simulink library "SimplusGT_2018b"  (R2018b)
settings: Solver=ode45  StartTime=0.0  StopTime=10.0  RelTol=1e-3
undefined symbols (not defined in the file): ang_r, Cf, DiscIntNeverNeededParam, initial, Lc, Lf, m, OtherInputs, P_dc, Sbase, t0, Tm_pu, Ts, V, Vbase, w_droop, w_i, w_pll, w_tau, w_v, Wbase, wc, wfil, x0, Ybase, Zbase
libraries: powerlib x224, SimplexPS_2015a x6, $bdroot x1
(part 1 of 5)
settings Model: Creator=admin_user  LastModifiedBy=yz34218
settings OptimizationCC: LifeSpan=inf
settings DebuggingCC: SFExecutionAtInitializationDiag=none
settings HardwareCC: ProdBitPerSizeT=32  ProdBitPerPtrDiffT=32  ProdWordSize=32  ProdHWDeviceType=Specified
settings SFSimCC: SimUseLocalCustomCode=off
settings RTWCC: RTWUseLocalCustomCode=off
settings CodeAppCC: StateflowObjectComments=on

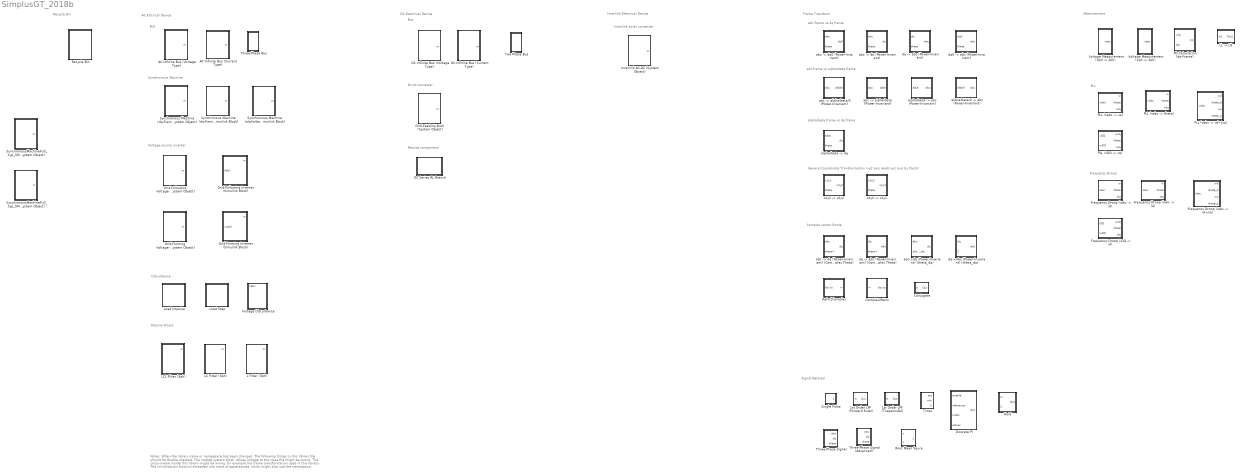
== system SimplusGT_2018b ==
  note: Notes:
      |
      | When the library name or namespace has been changed. The following things in this library file should be double checked.
      |
      | The matlab system block, whose linkage to the class file might be wrong.
      | The cross-invoke inside this library might be wrong, for example the frame transformation used in this library.
      | The initialization function embeded into mask of apparatuses, which might also use the namespace.
  note: Recycle Bin
  note: Interlink ac-dc converter
  note: Interlink Electrical Device
  note: Dc-dc converter:
  note: DC Electrical Device
  note: Passive Filters
  note: alpha/beta frame vs dq frame
  note: Frequency Droop
  note: PLL
  note: Complex vector frame
  note: abc frame vs alpha/beta frame
  note: abc frame vs dq frame
  note: Signal Related
  note: AC Elctrical Device
  note: Measurement
  note: Frame Transform
  note: Bus
  note: Synchronous Machine
  note: Voltage-source inverter
  note: Disturbance
  note: General Coordinate Transformation (xy2 axis leads xy1 axis by theta)
  note: Bus
  note: Passive component:
  1st Order LPF (Forward Euler) : Subsystem  mask{wc=wfil, Ts=Ts}
      mask prompts: wc "wc (rad/s), bandwidth"; Ts "Ts (s), sampling period"
  1st Order LPF (Trapezoidal) : Subsystem  mask{Ts=0, wc=0}
      mask prompts: Ts "Ts (s), sampling period"; wc "wc (rad/s), bandwidth"
  AC Infinite Bus (Current Type) : Subsystem  mask{Ts=Ts, Sbase=Sbase, Vbase=Vbase, Wbase=Wbase, id=1, iq=0, theta0=0, w=1}
      mask prompts: Ts "Ts (s), sampling period"; Sbase "Sbase (VA), base power"; Vbase "Vbase (V), base voltage"; Wbase "Wbase (rad/s), base angular frequency"; id "id (pu), d-axis current"; iq "iq (pu), q-axis current"; theta0 "theta0 (rad), initial angle"; w "w (pu), angular frequency"
  AC Infinite Bus (Voltage Type) : Subsystem  mask{Ts=Ts, Sbase=Sbase, Vbase=Vbase, Wbase=Wbase, vd=1, vq=0, theta0=0, w=Wbase, R=1e-30}
      mask prompts: Ts "Ts (s), samping period"; Sbase "Sbase (VA), power base"; Vbase "Vbase (V), voltage base"; Wbase "Wbase (rad/s), frequency base"; vd "vd (pu), d-axis voltage"; vq "vq (pu), q-axis voltage"; theta0 "theta0 (rad), initial angle"; w "w (rad/s), frequency"; R "R (Ohm), resistance"
  Complex2ReIm : Subsystem
  Conjugate : Subsystem
  DC Infinite Bus (Current Type) : Subsystem  mask{Ts=Ts, Sbase=Sbase, Vbase=Vbase, i=1, C=1e-9, R=1e-30}
      mask prompts: Ts "Ts (s), samping period"; Sbase "Sbase (VA), base power"; Vbase "Vbase (V), base voltage"; i "i (pu), current"; C "C (pu), capacitance"; R "R (pu), resistance"
  DC Infinite Bus (Voltage Type) : Subsystem  mask{Ts=Ts, Sbase=Sbase, Vbase=Vbase, v=1, R=1e-30}
      mask prompts: Ts "Ts (s), samping period"; Sbase "Sbase (VA), power base"; Vbase "Vbase (V), voltage base"; v "v (pu), voltage"; R "R (pu), resistance"
  DC Series RL Branch : Subsystem  mask{BranchType=RL, Resistance=0, Inductance=0}
      mask prompts: Resistance "Resistance (Ohms)"; Inductance "Inductance (H)"
      mask init:
      | if BranchType == 1
      |     set_param([gcb,'/Branch1'],'BranchType','R');
      |     set_param([gcb,'/Branch2'],'BranchType','R');
      | elseif BranchType == 2
      |     set_param([gcb,'/Branch1'],'BranchType','L');
      |     set_param([gcb,'/Branch2'],'BranchType','L');
      | elseif BranchType == 3
      |     set_param([gcb,'/Branch1'],'BranchType','RL');
      |     set_param([gcb,'/Branch2'],'BranchType','RL');
      | else
      |     error(['Error']);
      | end
      mask TypeOptions BranchType: R | L | RL
  Discrete PI : Subsystem  mask{Kp=wc, Ki=wc*wc/4, xmax=inf, xmin=-inf, Ts=Ts}
      mask prompts: Kp "Proportional Gain"; Ki "Integral Gain"; xmax "Upper Limit"; xmin "Lower Limit"; Ts "Sampling Time"
  "Frequency Droop (iDQ -> id)" : Subsystem  mask{Ts=Ts, Sbase=Sbase, Vbase=Vbase, Wbase=Wbase, m=m, w_tau=w_droop, theta0=0, i0=0, w0=1}
      mask prompts: Ts "Ts (s), sampling period"; Sbase "Sbase (VA), base power"; Vbase "Vbase (V), base voltage"; Wbase "Wbase (rad/s), base angular frequency"; m "m (pu), droop gain"; w_tau "w_tau (rad/s), low-pass filter bandwidth"; theta0 "theta0 (rad), initial angle"; i0 "i0 (pu), current setting point"; w0 "w0 (pu), frequency setting point"
  "Frequency Droop (iabc -> id)" : Subsystem  mask{Ts=Ts, Sbase=Sbase, Vbase=Vbase, Wbase=Wbase, m=m, w_tau=w_droop, theta0=0, i0=0, w0=1}
      mask prompts: Ts "Ts (s), samping period"; Sbase "Sbase (VA), base power"; Vbase "Vbase (V), base voltage"; Wbase "Wbase (rad/s), base angular frequency"; m "m (pu), droop gain"; w_tau "w_tau (rad/s), low-pass filter bandwidth"; theta0 "theta0 (rad), initial angle"; i0 "i0 (pu), current setting point"; w0 "w0 (pu), frequency setting point"
  "Frequency Droop (iabc -> id+jiq)" : Subsystem  mask{Ts=Ts, Sbase=Sbase, Vbase=Vbase, Wbase=Wbase, m=m, w_tau=w_droop, theta_d0=0, theta_q0=0, id0=0, iq0=0, wd0=1, wq0=0}
      mask prompts: Ts "Ts (s), sampling period"; Sbase "Sbase (VA), base power"; Vbase "Vbase (V), base voltage"; Wbase "Wbase (s), base frequency"; m "m (pu), droop gain"; w_tau "w_tau (pu), low-pass filter bandwidth"; theta_d0 "theta_d0 (rad/s), initial d-axis angle"; theta_q0 "theta_q0 (rad/s), initial q-axis angle"; id0 "id0 (pu), d-axis current setting point"; iq0 "iq0 (pu), q-axis current setting point"; wd0 "wd0 (pu), d-axis angular frequency setting point"; wq0 "wq0 (pu), q-axis angular frequency setting point"
  "Frequency Droop (iabc -> iq)" : Subsystem  mask{Ts=Ts, Sbase=Sbase, Vbase=Vbase, Wbase=Wbase, m=m, w_droop=w_droop, theta0=0, i0=0, w0=1}
      mask prompts: Ts "Ts (s), sampling period"; Sbase "Sbase (VA), base power"; Vbase "Vbase (V), base voltage"; Wbase "Wbase (rad/s), base angular frequency"; m "m (pu), droop gain"; w_droop "w_tau (rad/s), low-pass filter bandwidth"; theta0 "theta0 (rad), initial angle"; i0 "i0 (pu), current setting point"; w0 "w0 (pu), angular frequency setting point"
  Grid-Feeding Buck (System Object) : Subsystem  mask{Ts=Ts, Sbase=Sbase, Vbase=Vbase, ApparatusType=1010, ApparatusPara=[], PowerFlow=[], x0=x0, OtherInputs=[P_dc], DiscreMethod=Hybrid Trapezoidal, EnableInsideModification=off, DiscreDampingFlag=on, DiscreDampingValue=0, LinearizationTimes=1, DirectFeedthrough=off}
      mask prompts: Ts "Ts (s), samping period"; Sbase "Sbase (VA), power base"; Vbase "Vbase (V), voltage base"; ApparatusType "Apparatus type"; ApparatusPara "Apparatus parameters"; PowerFlow "Power flow parameters"; x0 "x0, initial states"; OtherInputs "Other inputs"; DiscreMethod "Discretization method"; EnableInsideModification "Enable inside modification"; DiscreDampingFlag "Enable discretization damping"; DiscreDampingValue "Discretization damping value"; LinearizationTimes "Linearization times"; DirectFeedthrough "Direct feedthrough"
      mask init:
      | SimplusGT.Simulink.DeviceMaskInitialization(EnableInsideModification,DiscreDampingFlag);
      mask TypeOptions DiscreMethod: Forward Euler | Hybrid Trapezoidal | Virtual Damping
      mask TypeOptions LinearizationTimes: 1 | 2
  Grid-Following Voltage-Source Inverter (dq-Frame System Object) : Subsystem  mask{Ts=Ts, Sbase=Sbase, Vbase=Vbase, Wbase=Wbase, ApparatusType=10, ApparatusPara=[], PowerFlow=[], x0=[0; 0; 0; 0; 2.5*Vbase; 0; 0; Wbase; 0], OtherInputs=[ang_r; P_dc], DiscreMethod=Hybrid Trapezoidal, EnableInsideModification=off, DiscreDampingFlag=on, DiscreDampingValue=0, LinearizationTimes=1, DirectFeedthrough=off}
      mask prompts: Ts "Ts (s), samping period"; Sbase "Sbase (VA), power base"; Vbase "Vbase (V), voltage base"; Wbase "Wbase (rad/s), frequency base"; ApparatusType "Apparatus type"; ApparatusPara "Apparatus parameters"; PowerFlow "Power flow parameters"; x0 "x0, initial states"; OtherInputs "Other inputs"; DiscreMethod "Discretization method"; EnableInsideModification "Enable inside modification"; DiscreDampingFlag "Enable discretization damping"; DiscreDampingValue "Discretization damping value"; LinearizationTimes "Linearization times"; DirectFeedthrough "Direct feedthrough"
      mask init:
      | SimplusGT.Simulink.DeviceMaskInitialization(EnableInsideModification,DiscreDampingFlag);
      mask TypeOptions DiscreMethod: Forward Euler | Hybrid Trapezoidal | Virtual Damping
      mask TypeOptions LinearizationTimes: 1 | 2
  Grid-Following Inverter (Simulink Block) : Subsystem  mask{Ts=Ts, Sbase=Sbase, Vbase=Vbase, Wbase=Wbase, w_i=w_i, w_pll=w_pll, w_tau=w_tau, Lf=Lf, Cf=Cf, Lc=Lc}
      mask prompts: Ts "Ts (s), sampling period"; Sbase "Sbase (VA), base power"; Vbase "Vbase (V), base voltage"; Wbase "Wbase (rad/s), base frequency"; w_i "w_i (rad/s), current-loop bandwidth"; w_pll "w_pll (rad/s), PLL bandwidth"; w_tau "w_tau (rad/s), PLL filter bandwidth"; Lf "Lf (pu), LCL filter"; Cf "Cf (pu), LCL filter"; Lc "Lc (pu), LCL filter"
  Grid-Forming Voltage-Source Inverter (dq-Frame System Object) : Subsystem  mask{Ts=Ts, Sbase=Sbase, Vbase=Vbase, Wbase=Wbase, ApparatusType=10, ApparatusPara=[], PowerFlow=[], x0=x0, OtherInputs=[ang_r; P_dc], DiscreMethod=Hybrid Trapezoidal, EnableInsideModification=off, DiscreDampingFlag=on, DiscreDampingValue=0, LinearizationTimes=1, DirectFeedthrough=off}
      mask prompts: Ts "Ts (s), samping period"; Sbase "Sbase (VA), power base"; Vbase "Vbase (V), voltage base"; Wbase "Wbase (rad/s), frequency base"; ApparatusType "Apparatus type"; ApparatusPara "Apparatus parameters"; PowerFlow "Power flow parameters"; x0 "x0, initial states"; OtherInputs "Other inputs"; DiscreMethod "Discretization method"; EnableInsideModification "Enable inside modification"; DiscreDampingFlag "Enable discretization damping"; DiscreDampingValue "Discretization damping value"; LinearizationTimes "Linearization times"; DirectFeedthrough "Direct feedthrough"
      mask init:
      | SimplusGT.Simulink.DeviceMaskInitialization(EnableInsideModification,DiscreDampingFlag);
      mask TypeOptions DiscreMethod: Forward Euler | Hybrid Trapezoidal | Virtual Damping
      mask TypeOptions LinearizationTimes: 1 | 2
  Grid-Forming Inverter (Simulink Block) : Subsystem  mask{Ts=Ts, Sbase=Sbase, Vbase=Vbase, Wbase=Wbase, w_i=w_i, w_v=w_v, w_droop=w_droop, m=m, Lf=Lf, Cf=Cf, Lc=Lc}
      mask prompts: Ts "Ts (s), sampling period"; Sbase "Sbase (VA), base power"; Vbase "Vbase (V), base voltage"; Wbase "Wbase (rad/s), base frequency"; w_i "w_i (rad/s), current-loop bandwidth"; w_v "w_v (rad/s), voltage-loop bandwidth"; w_droop "w_droop (rad/s), droop bandwidth"; m "m (pu), frequency droop gain"; Lf "Lf (pu), LCL filter"; Cf "Cf (pu), LCL filter"; Lc "Lc (pu), LCL filter"
  Hold : Subsystem
  Interlink AC-DC (System Object) : Subsystem  mask{Ts=Ts, Sbase=Sbase, Vbase=Vbase, Wbase=Wbase, ApparatusType=2000, ApparatusPara=[], PowerFlow=[], x0=x0, OtherInputs=OtherInputs, DiscreMethod=Hybrid Trapezoidal, EnableInsideModification=off, DiscreDampingFlag=on, DiscreDampingValue=0, LinearizationTimes=1, DirectFeedthrough=off}
      mask prompts: Ts "Ts (s), samping period"; Sbase "Sbase (VA), power base"; Vbase "Vbase (V), voltage base"; Wbase "Wbase (rad/s), frequency base"; ApparatusType "Apparatus type"; ApparatusPara "Apparatus parameters"; PowerFlow "Power flow parameters"; x0 "x0, initial states"; OtherInputs "Other inputs"; DiscreMethod "Discretization method"; EnableInsideModification "Enable inside modification"; DiscreDampingFlag "Enable discretization damping"; DiscreDampingValue "Discretization damping value"; LinearizationTimes "Linearization times"; DirectFeedthrough "Direct feedthrough"
      mask init:
      | SimplusGT.Simulink.DeviceMaskInitialInterlink(EnableInsideModification,DiscreDampingFlag);
      mask TypeOptions DiscreMethod: Forward Euler | Hybrid Trapezoidal | Virtual Damping
      mask TypeOptions LinearizationTimes: 1 | 2
  L Filter (3ph) : Subsystem  mask{Lf=Lf*Zbase/Wbase, Rf=1e-9}
      mask prompts: Lf "Lf (H)"; Rf "Rf (Ohm)"
  LC Filter (3ph) : Subsystem  mask{Lf=Lf*Zbase/Wbase, Rf=1e-9, Cf=Cf*Ybase/Wbase, Rd=1e-9}
      mask prompts: Lf "Lf (H)"; Rf "Rf (Ohm)"; Cf "Cf (F)"; Rd "Rd (Ohm)"
  LCL Filter (3ph) : Subsystem  mask{Lf=Lf*Zbase/Wbase, Rf=1e-9, Lc=Lc*Zbase/Wbase, Rc=1e-9, Cf=Cf*Ybase/Wbase, Rd=1e-20}
      mask prompts: Lf "Lf (H)"; Rf "Rf (Ohm)"; Lc "Lc (H)"; Rc "Rc (Ohm)"; Cf "Cf (F)"; Rd "Rd (Ohm)"
  "LL -> LN" : Subsystem
  Load Impulse : Subsystem  mask{t0=t0, dt=0.01, R=1*Zbase}
  Load Step : Subsystem  mask{t0=t0, R=1*Zbase, Reverse=0}
  "PLL (vDQ -> vq)" : Subsystem  mask{Ts=Ts, Vbase=Vbase, Wbase=Wbase, w_PLL=w_pll, w_tau=w_tau, theta0=0}
      mask prompts: Ts "Ts (s), sampling period"; Vbase "Vbase (V), base voltage"; Wbase "Wbase (rad/s), base angular frequency"; w_PLL "w_pll (rad/s), PLL bandwidth"; w_tau "w_tau (rad/s), low-pass filter bandwidth"; theta0 "theta0 (rad), initial angle"
  "PLL (vabc -> theta)" : Subsystem  mask{Ts=Ts, Wbase=Wbase, w_pll=w_pll, w_tau=w_tau, theta0=0}
      mask prompts: Ts "Ts (s), sampling period"; Wbase "Wbase (rad/s), frequency base"; w_pll "w_pll (rad/s), PLL bandwidth"; w_tau "w_tau (rad/s), low-pass filter bandwidth"; theta0 "theta0 (rad), initial angle"
  "PLL (vabc -> vd+jvq)" : Subsystem  mask{Ts=Ts, Vbase=Vbase, Wbase=Wbase, w_pll=w_pll, w_tau=w_tau, theta_d0=0, theta_q0=0}
      mask prompts: Ts "Ts (s), sampling period"; Vbase "Vbase (rad/s), base voltage"; Wbase "Wbase (rad/s), base frequency"; w_pll "w_pll (rad/s), PLL bandwidth"; w_tau "w_tau (rad/s), PLL filter"; theta_d0 "theta_d0 (rad), initial d-axis angle"; theta_q0 "theta_q0 (rad), initial q-axis angle"
  "PLL (vabc -> vq)" : Subsystem  mask{Ts=Ts, Vbase=Vbase, Wbase=Wbase, w_pll=w_pll, w_tau=w_tau, theta0=0}
      mask prompts: Ts "Ts (s), sampling period"; Vbase "Vbase (V), base voltage"; Wbase "Wbase (rad/s), base angular frequency"; w_pll "w_pll (rad/s), PLL bandwidth"; w_tau "w_tau (rad/s), low-pass filter bandwidth"; theta0 "theta0 (rad), initial angle"
  PQ Calculation (dq-Frame) : Subsystem
  ReIm2Complex : Subsystem
  Recycle Bin : Subsystem
  Root Mean Squre : Subsystem
  Single Pulse : Subsystem  mask{t0=0, dt=0.1, Am=1}
      mask prompts: t0 "t0 (s), starting time"; dt "dt (s), pulse width"; Am "Am, pulse amplitude"
  Synchronous Machine (alpha/beta-Frame) (Simulink Block) : Subsystem  mask{Ts=Ts, Sbase=Sbase, Vbase=Vbase, Wbase=Wbase, R=0.01, L=0.3, J=2*3.5, D=10, psi_f=1.1229, Tm=-10.890, w0=1, theta0=0}
      mask prompts: Ts "Ts (s), samping period"; Sbase "Sbase (VA), power base"; Vbase "Vbase (V), voltage base"; Wbase "Wbase (rad/s), frequency base"; R "R (pu), stator resistance"; L "L (pu), stator inductance"; J "J (pu), rotor inertia"; D "D (pu), damping torque coefficient"; psi_f "psi_f (pu), field flux linkage"; Tm "Tm (pu), mechanical torque"; w0 "w0 (pu), initial rotor speed"; theta0 "theta0 (rad), initial rotor angle"
  Synchronous Machine (dq-Frame System Object) : Subsystem  mask{Ts=Ts, Sbase=Sbase, Vbase=Vbase, Wbase=Wbase, ApparatusType=0, ApparatusPara=[], PowerFlow=[], x0=[0;0;Wbase;0], OtherInputs=[Tm_pu/Wbase;0], DiscreMethod=Hybrid Trapezoidal, EnableInsideModification=off, DiscreDampingFlag=on, DiscreDampingValue=0, LinearizationTimes=1, DirectFeedthrough=off}
      mask prompts: Ts "Ts (s), samping period"; Sbase "Sbase (VA), power base"; Vbase "Vbase (V), voltage base"; Wbase "Wbase (rad/s), frequency base"; ApparatusType "Apparatus type"; ApparatusPara "Apparatus parameters"; PowerFlow "Power flow paramters"; x0 "x0, initial states"; OtherInputs "Other inputs"; DiscreMethod "Discrerization method"; EnableInsideModification "Enable inside modification"; DiscreDampingFlag "Enable discretization damping"; DiscreDampingValue "Discretization damping value"; LinearizationTimes "Linearization times"; DirectFeedthrough "Direct feedthrough"
      mask init:
      | SimplusGT.Simulink.DeviceMaskInitialization(EnableInsideModification,DiscreDampingFlag);
      mask TypeOptions DiscreMethod: Forward Euler | Hybrid Trapezoidal | Virtual Damping
      mask TypeOptions LinearizationTimes: 1 | 2
  Synchronous Machine (dq-Frame) (Simulink Block) : Subsystem  mask{Ts=Ts, Sbase=Sbase, Vbase=Vbase, Wbase=Wbase, R=0.01, L=0.3, J=2*3.5, D=10, psi_f=1.1229, Tm=-10.890, w0=1, theta0=0}
      mask prompts: Ts "Ts (s), samping period"; Sbase "Sbase (VA), power base"; Vbase "Vbase (V), voltage base"; Wbase "Wbase (rad/s), frequency base"; R "R (pu), stator resistance"; L "L (pu), stator inductance"; J "J (pu), rotor inertia"; D "D (pu), damping torque coefficient"; psi_f "psi_f (pu), field flux linkage"; Tm "Tm (pu), mechanical torque"; w0 "w0 (pu), intial rotor speed"; theta0 "theta0 (rad), initial rotor angle"
  SynchronousMachineFull_Cyp_SMAVR (dq-Frame System Object) : Subsystem  mask{Ts=Ts, Sbase=Sbase, Vbase=Vbase, Wbase=Wbase, ApparatusType=0, ApparatusPara=[], PowerFlow=[], x0=[0;0;Wbase;0], OtherInputs=[Tm_pu/Wbase;0], DiscreMethod=Hybrid Trapezoidal, EnableInsideModification=off, DiscreDampingFlag=on, DiscreDampingValue=0, LinearizationTimes=1, DirectFeedthrough=off}
      mask prompts: Ts "Ts (s), samping period"; Sbase "Sbase (VA), power base"; Vbase "Vbase (V), voltage base"; Wbase "Wbase (rad/s), frequency base"; ApparatusType "Apparatus type"; ApparatusPara "Apparatus parameters"; PowerFlow "Power flow paramters"; x0 "x0, initial states"; OtherInputs "Other inputs"; DiscreMethod "Discrerization method"; EnableInsideModification "Enable inside modification"; DiscreDampingFlag "Enable discretization damping"; DiscreDampingValue "Discretization damping value"; LinearizationTimes "Linearization times"; DirectFeedthrough "Direct feedthrough"
      mask init:
      | SimplusGT.Simulink.DeviceMaskInitialization(EnableInsideModification,DiscreDampingFlag);
      mask TypeOptions DiscreMethod: Forward Euler | Hybrid Trapezoidal | Virtual Damping
      mask TypeOptions LinearizationTimes: 1 | 2
  SynchronousMachineFull_Cyp_SMAVRPSSGOV (dq-Frame System Object) : Subsystem  mask{Ts=Ts, Sbase=Sbase, Vbase=Vbase, Wbase=Wbase, ApparatusType=0, ApparatusPara=[], PowerFlow=[], x0=[0;0;Wbase;0], OtherInputs=[Tm_pu/Wbase;0], DiscreMethod=Hybrid Trapezoidal, EnableInsideModification=off, DiscreDampingFlag=on, DiscreDampingValue=0, LinearizationTimes=1, DirectFeedthrough=off}
      mask prompts: Ts "Ts (s), samping period"; Sbase "Sbase (VA), power base"; Vbase "Vbase (V), voltage base"; Wbase "Wbase (rad/s), frequency base"; ApparatusType "Apparatus type"; ApparatusPara "Apparatus parameters"; PowerFlow "Power flow paramters"; x0 "x0, initial states"; OtherInputs "Other inputs"; DiscreMethod "Discrerization method"; EnableInsideModification "Enable inside modification"; DiscreDampingFlag "Enable discretization damping"; DiscreDampingValue "Discretization damping value"; LinearizationTimes "Linearization times"; DirectFeedthrough "Direct feedthrough"
      mask init:
      | SimplusGT.Simulink.DeviceMaskInitialization(EnableInsideModification,DiscreDampingFlag);
      mask TypeOptions DiscreMethod: Forward Euler | Hybrid Trapezoidal | Virtual Damping
      mask TypeOptions LinearizationTimes: 1 | 2
  Three-Phase Bus : Subsystem  mask{Vbase=1, Sbase=1}
  Three-Phase Signal : Subsystem  mask{Ts=Ts, ud=1, uq=0, w=Wbase, theta0=0}
      mask prompts: Ts "Ts (s), sampling period"; w "w (rad/s), angular frequency"; theta0 "theta0 (rad), initial angle"
  Three-Phase Signal (Advanced) : Subsystem  mask{Ts=Ts, ud=1, uq=0, w=Wbase, theta0=0, enable_freq_step=0, ratio_freq_step=0, time_freq_step=99}
      mask prompts: Ts "Ts (s), sampling period"; w "w (rad/s), angular frequency"; theta0 "theta0 (rad), initial angle"; enable_freq_step "enable: frequency step"; ratio_freq_step "ratio: frequency step"; time_freq_step "time (s): frequency step"
  Timer : Subsystem  mask{Ts=0}
      mask prompts: Ts "Ts (s), samping period"
  Two-Phase Bus : Subsystem  mask{Vbase=1, Sbase=1}
  "Voltage Measurement (2ph -> 3ph)" : Subsystem
  "Voltage Measurement (3ph -> 3ph)" : Subsystem
  Voltage Disturbance : Subsystem  mask{Vbase=Vbase}
  "abc -> alpha/beta (Power-Invariant)" : Subsystem
  "abc -> alpha/beta/0 (Power-Invariant)" : Subsystem
  "abc -> dq (Power-Invariant)" : Subsystem
  "abc -> dq (Power-Invariant) (Complex Theta)" : Subsystem
  "abc -> dq0 (Power-Invariant)" : Subsystem
  abc->dq (Power-Invariant) (theta_dq) : Subsystem
  "alpha/beta -> abc (Power-Invariant)" : Subsystem
  "alpha/beta -> dq" : Subsystem
  "alpha/beta/0 -> abc (Power-Invariant)" : Subsystem
  "dq -> abc (Power-Invariant)" : Subsystem
  "dq -> abc (Power-Invariant) (Complex Theta)" : Subsystem
  dq->abc (Power-Invariant) (theta_dq) : Subsystem
  "dq0 -> abc (Power-Invariant)" : Subsystem
  "x1y1 -> x2y2" : Subsystem
  "x2y2 -> x1y1" : Subsystem

== system SimplusGT_2018b/1st Order LPF (Forward Euler) ==
  note: 1st order digital low pass filter
      |
      | Author(s): Yitong Li
      |
      | Notes:
      |
      | This is the z-domain 1st-order LPF, wc*Ts/(wc*Ts + z-1), which can be obtained by simply applying the Euler transform (i.e., s -> (z-1)/Ts) to the s-domain 1st-order LPF, 1/(1 + s/wc), where wc is the bandwidth of the LPF.
  In : Inport
  Euler : DiscreteTransferFcn  Numerator=wc*Ts  Denominator=[1 ((wc*Ts)-1)]  SampleTime=Ts
  Out : Outport
  wires:
  In/1 -> Euler/1
  Euler/1 -> Out/1

== system SimplusGT_2018b/1st Order LPF (Trapezoidal) ==
  note: 1st order digital low pass filter
      |
      | Author(s): Yitong Li
      |
      | Notes:
      |
      | The trapezoidal discretization is used.
  In : Inport
  Trapezoidal : DiscreteTransferFcn  Numerator=[wc*Ts wc*Ts]  Denominator=[wc*Ts+2 wc*Ts-2]  SampleTime=Ts
  Out : Outport
  wires:
  In/1 -> Trapezoidal/1
  Trapezoidal/1 -> Out/1

== system SimplusGT_2018b/AC Infinite Bus (Current Type) ==
  note: Current-type infinite bus.
      |
      | Author(s): Yitong Li
      |
      | Notes:
      |
      | Current-type means the infinite bus is a current source rather than a voltage source.
      |
      | The system is in source convention.
  note: Auxiliary
  note: Electrical Circuit
  Bus Creator : BusCreator  Inputs=7
  Constant : Constant  Value=[id iq]
  Constant1 : Constant  Value=w
  Constant2 : Constant  Value=theta0
  Constant3 : Constant  Value=2*pi
  Controlled Current Source : powerlib/Electrical Sources/Controlled Current Source  Initialize=on  Source_Type=AC  Amplitude=0  Phase=0  Frequency=0  Measurements=None
  Controlled Current Source1 : powerlib/Electrical Sources/Controlled Current Source  Initialize=on  Source_Type=AC  Amplitude=0  Phase=0  Frequency=0  Measurements=None
  Controlled Current Source2 : powerlib/Electrical Sources/Controlled Current Source  Initialize=on  Source_Type=AC  Amplitude=0  Phase=0  Frequency=0  Measurements=None
  Demux : Demux  Outputs=3
  Discrete-Time Integrator : DiscreteIntegrator  IntegratorMethod=Integration: Trapezoidal  InitialConditionSource=external  SampleTime=-1  ICPrevOutput=DiscIntNeverNeededParam  ICPrevScaledInput=DiscIntNeverNeededParam
  Gain : Gain  Gain=Wbase
  Gain1 : Gain  Gain=Sbase/Vbase
  Gain3 : Gain  Gain=1/Vbase
  Math Function1 : Math  Operator=mod  SaturateOnIntegerOverflow=on
  Mux : Mux  Inputs=3
  PQ Calculation (dq-Frame) : Subsystem  AncestorBlock=|
      | SimplusGT/PQ Calculation
      | (dq-Frame)
  Three-Phase Parallel RLC Branch : powerlib/Elements/Three-Phase Parallel RLC Branch  LConnTagsString=A|B|C  RConnTagsString=A|B|C  BranchType=C  Resistance=1  Inductance=1e-3  Capacitance=1e-9  Measurements=None
      settings: SourceProductName=Simscape Power Systems  SourceProductBaseCode=PS
  Voltage Measurement : powerlib/Measurements/Voltage Measurement  PhasorSimulation=off  OutputType=Complex  PSBequivalent=0
  Voltage Measurement1 : powerlib/Measurements/Voltage Measurement  PhasorSimulation=off  OutputType=Complex  PSBequivalent=0
  Voltage Measurement2 : powerlib/Measurements/Voltage Measurement  PhasorSimulation=off  OutputType=Complex  PSBequivalent=0
  "abc -> dq (Power-Invariant)" : Subsystem  AncestorBlock=|
      | SimplusGT/abc -> dq
      | (Power-Invariant)
  "dq -> abc (Power-Invariant)" : Subsystem  AncestorBlock=|
      | SimplusGT/dq -> abc
      | (Power-Invariant)
  a : PMIOPort  Side=Left
  b : PMIOPort  Port=2  Side=Left
  c : PMIOPort  Port=3  Side=Left
  n : PMIOPort  Port=4  Side=Left
  m : Outport
  wires:
  Demux/3 -> Controlled Current Source2/1
  [v_dq] -> Bus Creator/1  "v_dq"
  "dq -> abc (Power-Invariant)"/1(abc) -> [i_abc]
  [pq] -> Bus Creator/7  "pq"
  [theta] -> "abc -> dq (Power-Invariant)"/2(theta)
  Demux/2 -> Controlled Current Source1/1
  "abc -> dq (Power-Invariant)"/1(dq) -> [v_dq]
  Bus Creator/1 -> m/1
  Constant1/1 -> Gain/1, [w]
  [i_dq] -> Bus Creator/2  "i_dq"
  [w] -> Bus Creator/5  "w"
  Gain1/1 -> Demux/1
  Mux/1 -> Gain3/1
  [v_abc] -> "abc -> dq (Power-Invariant)"/1(abc)
  PQ Calculation (dq-Frame)/1(pq) -> [pq]
  [i_abc] -> Gain1/1
  Constant/1 -> "dq -> abc (Power-Invariant)"/1(dq), [i_dq]
  Demux/1 -> Controlled Current Source/1
  Math Function1/1 -> "dq -> abc (Power-Invariant)"/2(theta), [theta]
  Constant2/1 -> Discrete-Time Integrator/2
  Gain3/1 -> [v_abc]
  [theta] -> Bus Creator/6  "theta"
  [i_abc] -> Bus Creator/4  "i_abc"
  Constant3/1 -> Math Function1/2
  Discrete-Time Integrator/1 -> Math Function1/1
  [v_abc] -> Bus Creator/3  "v_abc"
  [v_dq] -> PQ Calculation (dq-Frame)/1(vdq)  "v_dq"
  [i_dq] -> PQ Calculation (dq-Frame)/2(idq)  "i_dq"
  Voltage Measurement/1 -> Mux/1
  Voltage Measurement1/1 -> Mux/2
  Voltage Measurement2/1 -> Mux/3
  Gain/1 -> Discrete-Time Integrator/1
  connections:
  b/RConn1 -- Three-Phase Parallel RLC Branch/LConn2 -- Voltage Measurement1/LConn1 -- Controlled Current Source1/RConn1
  c/RConn1 -- Three-Phase Parallel RLC Branch/LConn3 -- Controlled Current Source2/RConn1 -- Voltage Measurement2/LConn1
  n/RConn1 -- Three-Phase Parallel RLC Branch/RConn1 -- Three-Phase Parallel RLC Branch/RConn3 -- Three-Phase Parallel RLC Branch/RConn2 -- Voltage Measurement2/LConn2 -- Controlled Current Source2/LConn1 -- Voltage Measurement1/LConn2 -- Controlled Current Source1/LConn1 -- Voltage Measurement/LConn2 -- Controlled Current Source/LConn1
  a/RConn1 -- Three-Phase Parallel RLC Branch/LConn1 -- Controlled Current Source/RConn1 -- Voltage Measurement/LConn1

== system SimplusGT_2018b/AC Infinite Bus (Voltage Type) ==
  note: Model for voltage-type infinite bus.
      |
      | Author(s): Yitong Li
      |
      | The system is in load convention.
  note: Electrical Circuit
  note: Auxiliary
  Bus Creator : BusCreator  Inputs=7
  Constant : Constant  Value=[vd vq]
  Constant1 : Constant  Value=w
  Constant2 : Constant  Value=theta0
  Constant3 : Constant  Value=2*pi
  Demux : Demux  Outputs=3
  Discrete-Time Integrator : DiscreteIntegrator  IntegratorMethod=Integration: Trapezoidal  InitialConditionSource=external  SampleTime=-1  ICPrevOutput=DiscIntNeverNeededParam  ICPrevScaledInput=DiscIntNeverNeededParam
  Gain1 : Gain  Gain=Vbase
  Gain2 : Gain  Gain=1/Wbase
  Gain3 : Gain  Gain=1/(Sbase/Vbase)
  Math Function1 : Math  Operator=mod  SaturateOnIntegerOverflow=on
  Mux : Mux  Inputs=3
  PQ Calculation (dq-Frame)1 : Subsystem  AncestorBlock=|
      | SimplusGT/PQ Calculation
      | (dq-Frame)
  Ra : powerlib/Elements/Series RLC Branch  LConnTagsString=__new0  RConnTagsString=__new0  BranchType=R  Resistance=R  Inductance=1e-3  SetiL0=off  InitialCurrent=0  Capacitance=1e-6  Setx0=off  InitialVoltage=0  Measurements=None
  Rb : powerlib/Elements/Series RLC Branch  LConnTagsString=__new0  RConnTagsString=__new0  BranchType=R  Resistance=R  Inductance=1e-3  SetiL0=off  InitialCurrent=0  Capacitance=1e-6  Setx0=off  InitialVoltage=0  Measurements=None
  Rc : powerlib/Elements/Series RLC Branch  LConnTagsString=__new0  RConnTagsString=__new0  BranchType=R  Resistance=R  Inductance=1e-3  SetiL0=off  InitialCurrent=0  Capacitance=1e-6  Setx0=off  InitialVoltage=0  Measurements=None
  "abc -> dq (Power-Invariant)1" : Subsystem  AncestorBlock=|
      | SimplusGT/abc -> dq
      | (Power-Invariant)
  "dq -> abc (Power-Invariant)1" : Subsystem  AncestorBlock=|
      | SimplusGT/dq -> abc
      | (Power-Invariant)
  ia : powerlib/Measurements/Current Measurement  PhasorSimulation=off  OutputType=Complex  PSBequivalent=0
  ib : powerlib/Measurements/Current Measurement  PhasorSimulation=off  OutputType=Complex  PSBequivalent=0
  ic : powerlib/Measurements/Current Measurement  PhasorSimulation=off  OutputType=Complex  PSBequivalent=0
  va : powerlib/Electrical Sources/Controlled Voltage Source  Initialize=on  Source_Type=AC  Amplitude=0  Phase=0  Frequency=0  Measurements=None
  vb : powerlib/Electrical Sources/Controlled Voltage Source  Initialize=on  Source_Type=AC  Amplitude=0  Phase=0  Frequency=0  Measurements=None
  vc : powerlib/Electrical Sources/Controlled Voltage Source  Initialize=on  Source_Type=AC  Amplitude=0  Phase=0  Frequency=0  Measurements=None
  a : PMIOPort  Side=Left
  b : PMIOPort  Port=2  Side=Left
  c : PMIOPort  Port=3  Side=Left
  n : PMIOPort  Port=4  Side=Left
  m : Outport
  wires:
  [v_abc] -> Gain1/1
  Demux/1 -> va/1
  Demux/2 -> vb/1
  Demux/3 -> vc/1
  Math Function1/1 -> "dq -> abc (Power-Invariant)1"/2(theta), [theta]
  Constant2/1 -> Discrete-Time Integrator/2
  Constant1/1 -> Discrete-Time Integrator/1, [w]
  "dq -> abc (Power-Invariant)1"/1(abc) -> [v_abc]
  Constant3/1 -> Math Function1/2
  Constant/1 -> "dq -> abc (Power-Invariant)1"/1(dq), [v_dq]
  Discrete-Time Integrator/1 -> Math Function1/1
  [v_dq] -> Bus Creator/1  "v_dq"
  [i_abc] -> Bus Creator/4  "i_abc"
  [w] -> Gain2/1  "w"
  [v_abc] -> Bus Creator/3  "v_abc"
  Gain2/1 -> Bus Creator/5  "w"
  [i_dq] -> Bus Creator/2  "i_dq"
  Bus Creator/1 -> m/1
  [theta] -> Bus Creator/6  "theta"
  ia/1 -> Mux/1
  ib/1 -> Mux/2
  ic/1 -> Mux/3
  [i_abc] -> "abc -> dq (Power-Invariant)1"/1(abc)
  [theta] -> "abc -> dq (Power-Invariant)1"/2(theta)
  "abc -> dq (Power-Invariant)1"/1(dq) -> [i_dq]
  Gain1/1 -> Demux/1
  Mux/1 -> Gain3/1
  Gain3/1 -> [i_abc]
  [v_dq] -> PQ Calculation (dq-Frame)1/1(vdq)  "v_dq"
  [i_dq] -> PQ Calculation (dq-Frame)1/2(idq)  "i_dq"
  PQ Calculation (dq-Frame)1/1(pq) -> [pq]
  [pq] -> Bus Creator/7  "pq"
  connections:
  vc/LConn1 -- n/RConn1 -- va/LConn1 -- vb/LConn1
  ia/RConn1 -- va/RConn1
  ib/RConn1 -- vb/RConn1
  ic/RConn1 -- vc/RConn1
  Ra/RConn1 -- ia/LConn1
  Ra/LConn1 -- a/RConn1
  ib/LConn1 -- Rb/RConn1
  Rb/LConn1 -- b/RConn1
  Rc/RConn1 -- ic/LConn1
  Rc/LConn1 -- c/RConn1

== system SimplusGT_2018b/Complex2ReIm ==
  +- : Inport
  ->Im : Fcn  Expr=(u[1]-u[2])/2/1i
  ->Re : Fcn  Expr=(u[1]+u[2])/2
  Mux : Mux  Inputs=2
  Re Im : Outport
  wires:
  +-/1 -> ->Im/1, ->Re/1
  Mux/1 -> Re Im/1
  ->Re/1 -> Mux/1
  ->Im/1 -> Mux/2

== system SimplusGT_2018b/Conjugate ==
  note: Conjugate
      |
      | Author(s): Yitong Li
  In : Inport
  Complex to Real-Imag : ComplexToRealImag
  Gain : Gain  Gain=-1
  Real-Imag to Complex : RealImagToComplex
  Out : Outport
  wires:
  Complex to Real-Imag/1 -> Real-Imag to Complex/1
  Complex to Real-Imag/2 -> Gain/1
  Real-Imag to Complex/1 -> Out/1
  Gain/1 -> Real-Imag to Complex/2
  In/1 -> Complex to Real-Imag/1

== system SimplusGT_2018b/DC Infinite Bus (Current Type) ==
  note: Model for current-type dc infinite bus.
      |
      | Author(s): Yitong Li
  Bus Creator : BusCreator  Inputs=3
  Constant4 : Constant  Value=i
  Controlled Current Source : powerlib/Electrical Sources/Controlled Current Source  Initialize=on  Source_Type=AC  Amplitude=0  Phase=0  Frequency=0  Measurements=None
  Gain1 : Gain  Gain=1/Vbase
  Gain3 : Gain  Gain=Sbase/Vbase
  Product : Product
  RC : powerlib/Elements/Series RLC Branch  LConnTagsString=__new0  RConnTagsString=__new0  BranchType=RC  Resistance=R*V^2/Sbase  Inductance=1e-3  SetiL0=off  InitialCurrent=0  Capacitance=C/(2*pi*50)*Sbase/Vbase^2  Setx0=off  InitialVoltage=0  Measurements=None
  Voltage Measurement : powerlib/Measurements/Voltage Measurement  PhasorSimulation=off  OutputType=Complex  PSBequivalent=0
  + : PMIOPort  Side=Left
  - : PMIOPort  Port=2  Side=Left
  m : Outport
  wires:
  Constant4/1 -> [i], Gain3/1, Product/2
  [v] -> Bus Creator/1  "v"
  [i] -> Bus Creator/2  "i"
  Bus Creator/1 -> m/1
  Gain3/1 -> Controlled Current Source/1
  Gain1/1 -> Product/1, [v]
  [p] -> Bus Creator/3  "p"
  Product/1 -> [p]
  Voltage Measurement/1 -> Gain1/1
  connections:
  -/RConn1 -- RC/RConn1 -- Voltage Measurement/LConn2 -- Controlled Current Source/LConn1
  Controlled Current Source/RConn1 -- +/RConn1 -- RC/LConn1 -- Voltage Measurement/LConn1

== system SimplusGT_2018b/DC Infinite Bus (Voltage Type) ==
  note: Model for voltage-type dc infinite bus.
      |
      | Author(s): Yitong Li
  Bus Creator : BusCreator  Inputs=3
  Constant4 : Constant  Value=v
  Gain1 : Gain  Gain=Vbase
  Gain3 : Gain  Gain=1/(Sbase/Vbase)
  Product : Product
  R : powerlib/Elements/Series RLC Branch  LConnTagsString=__new0  RConnTagsString=__new0  BranchType=R  Resistance=R*Vbase^2/Sbase  Inductance=1e-3  SetiL0=off  InitialCurrent=0  Capacitance=1e-6  Setx0=off  InitialVoltage=0  Measurements=None
  i : powerlib/Measurements/Current Measurement  PhasorSimulation=off  OutputType=Complex  PSBequivalent=0
  v : powerlib/Electrical Sources/Controlled Voltage Source  Initialize=on  Source_Type=AC  Amplitude=0  Phase=0  Frequency=0  Measurements=None
  + : PMIOPort  Side=Left
  - : PMIOPort  Port=2  Side=Left
  m : Outport
  wires:
  Constant4/1 -> Product/2, [v], Gain1/1
  [v] -> Bus Creator/1  "v"
  [i] -> Bus Creator/2  "i"
  Bus Creator/1 -> m/1
  Gain1/1 -> v/1
  i/1 -> Gain3/1
  Gain3/1 -> Product/1, [i]
  [p] -> Bus Creator/3  "p"
  Product/1 -> [p]
  connections:
  v/LConn1 -- -/RConn1
  i/RConn1 -- v/RConn1
  R/RConn1 -- i/LConn1
  R/LConn1 -- +/RConn1

== system SimplusGT_2018b/DC Series RL Branch ==
  Branch1 : powerlib/Elements/Series RLC Branch  LConnTagsString=__new0  RConnTagsString=__new0  BranchType=RL  Resistance=Resistance/2  Inductance=Inductance/2  SetiL0=off  InitialCurrent=0  Capacitance=1e-6  Setx0=off  InitialVoltage=0  Measurements=None
  Branch2 : powerlib/Elements/Series RLC Branch  LConnTagsString=__new0  RConnTagsString=__new0  BranchType=RL  Resistance=Resistance/2  Inductance=Inductance/2  SetiL0=off  InitialCurrent=0  Capacitance=1e-6  Setx0=off  InitialVoltage=0  Measurements=None
  a+ : PMIOPort  Side=Left
  a- : PMIOPort  Port=2  Side=Right
  b+ : PMIOPort  Port=3  Side=Left
  b- : PMIOPort  Port=4  Side=Right
  connections:
  Branch1/RConn1 -- a-/RConn1
  Branch2/LConn1 -- b+/RConn1
  Branch2/RConn1 -- b-/RConn1
  Branch1/LConn1 -- a+/RConn1

== system SimplusGT_2018b/Discrete PI ==
  note: Digital PI controller
      |
      | Author(s): Yitong Li
  enable : Inport
  reference : Inport  Port=2
  initial : Inport  Port=3
  actual : Inport  Port=4
  Discrete-Time Integrator : DiscreteIntegrator  gainval=1  ExternalReset=rising  InitialConditionSource=external  InitialCondition=initial  SampleTime=Ts  LimitOutput=on  UpperSaturationLimit=xmax  LowerSaturationLimit=xmin  ICPrevOutput=DiscIntNeverNeededParam  ICPrevScaledInput=DiscIntNeverNeededParam
  Ierror : Sum  Inputs=+-
  Ki : Gain  Gain=Ki  SaturateOnIntegerOverflow=on  OutDataTypeStr=Inherit: Same as input  ParamDataTypeStr=Inherit: Same as input
  Kp : Gain  Gain=Kp  SaturateOnIntegerOverflow=on  OutDataTypeStr=Inherit: Same as input  ParamDataTypeStr=Inherit: Same as input
  Perror : Sum  Inputs=-+
  Product : Product  RndMeth=Zero
  Product1 : Product  RndMeth=Zero
  Saturation : Saturate  UpperLimit=xmax  LowerLimit=xmin
  Sum1 : Sum  SaturateOnIntegerOverflow=on
  Out : Outport
  wires:
  Saturation/1 -> Out/1
  Sum1/1 -> Saturation/1
  Ki/1 -> Discrete-Time Integrator/1
  Kp/1 -> Sum1/1
  Discrete-Time Integrator/1 -> Sum1/2
  enable/1 -> Discrete-Time Integrator/2, Product/2, Product1/2
  initial/1 -> Discrete-Time Integrator/3
  reference/1 -> Perror/2, Ierror/1
  actual/1 -> Ierror/2, Perror/1
  Perror/1 -> Product/1
  Product/1 -> Kp/1
  Ierror/1 -> Product1/1
  Product1/1 -> Ki/1

== system SimplusGT_2018b/Frequency Droop (iDQ -> id) ==
  note: Measurement
  note: Frequency droop controller
      |
      | Author(s): Yitong Li
      |
      | Notes:
      |
      | vq is fed into the PI controller of the PLL.
      |
      | This control assumes the input current is in DQ frame, which is the common electrical frame. It is not a practical frequency droop control which uses iabc or PQ as the input. But this controller is useful in research.
  iDQ : Inport
  wDQ : Inport  Port=2
  Constant : Constant  Value=w0
  Constant2 : Constant  Value=theta0
  Constant4 : Constant  Value=2*pi
  Constant6 : Constant  Value=i0
  Demux1 : Demux  Outputs=2
  Discrete-Time Integrator : DiscreteIntegrator  SampleTime=Ts  ICPrevOutput=DiscIntNeverNeededParam  ICPrevScaledInput=DiscIntNeverNeededParam
  Filter p : DiscreteTransferFcn  Numerator=w_tau*Ts  Denominator=[1 ((w_tau*Ts)-1)]  SampleTime=Ts
  Gain1 : Gain  Gain=1/(Sbase/Vbase)
  Gain2 : Gain  Gain=m
  Gain3 : Gain  Gain=Wbase
  Gain4 : Gain  Gain=1/Wbase
  Gain5 : Gain  Gain=1/pi
  Math Function1 : Math  Operator=mod  SaturateOnIntegerOverflow=on
  Mux : Mux  Inputs=2
  Scope : Scope  NumInputPorts=4
  Sum : Sum
  Sum1 : Sum
  Sum2 : Sum  Inputs=+-
  Sum3 : Sum  Inputs=+-
  "x1y1 -> x2y2" : Subsystem  AncestorBlock=SimplusGT/x1y1 -> x2y2
  wdq : Outport
  theta : Outport  Port=2
  idq : Outport  Port=3
  wires:
  Gain1/1 -> Filter p/1
  Math Function1/1 -> "x1y1 -> x2y2"/2(theta), theta/1, [theta]
  Constant6/1 -> Sum2/1
  Constant/1 -> Sum/2
  [iq] -> Scope/2  "iq"
  Constant2/1 -> Sum1/2, [theta0]
  Constant4/1 -> Math Function1/2
  Gain2/1 -> Sum/1
  Sum1/1 -> Math Function1/1
  Discrete-Time Integrator/1 -> Sum1/1
  Gain5/1 -> Scope/4
  iDQ/1 -> "x1y1 -> x2y2"/1(x1y1)
  "x1y1 -> x2y2"/1(x2y2) -> idq/1, Demux1/1
  [theta0] -> Mux/1  "theta"
  Gain3/1 -> wdq/1, [w], Discrete-Time Integrator/1
  Sum2/1 -> Gain2/1
  Mux/1 -> Gain5/1  "theta"
  Demux1/1 -> Gain1/1, [id]  "id"
  [w] -> Gain4/1  "w"
  Gain4/1 -> Scope/3
  [theta] -> Mux/2  "theta"
  [id] -> Scope/1  "id"
  Filter p/1 -> Sum2/2
  Demux1/2 -> [iq]
  Sum/1 -> Sum3/1
  Sum3/1 -> Gain3/1
  wDQ/1 -> Sum3/2

== system SimplusGT_2018b/Frequency Droop (iabc -> id) ==
  note: Measurement
  note: id-frequency droop controller
      |
      | Author(s): Yitong Li
      |
      | Notes:
      |
      | The current reference should be in source convention.
      |
      | It is a id-frequency droop controller rather than a power-frequency droop controller.
  iabc : Inport
  Constant : Constant  Value=w0
  Constant2 : Constant  Value=theta0
  Constant4 : Constant  Value=2*pi
  Constant6 : Constant  Value=i0
  Demux1 : Demux  Outputs=2
  Discrete-Time Integrator : DiscreteIntegrator  SampleTime=Ts  ICPrevOutput=DiscIntNeverNeededParam  ICPrevScaledInput=DiscIntNeverNeededParam
  Filter p : DiscreteTransferFcn  Numerator=w_tau*Ts  Denominator=[1 ((w_tau*Ts)-1)]  SampleTime=Ts
  Gain1 : Gain  Gain=1/(Sbase/Vbase)
  Gain2 : Gain  Gain=m
  Gain3 : Gain  Gain=Wbase
  Gain4 : Gain  Gain=1/Wbase
  Gain5 : Gain  Gain=1/pi
  Math Function1 : Math  Operator=mod  SaturateOnIntegerOverflow=on
  Mux : Mux  Inputs=2
  Scope : Scope  NumInputPorts=4
  Sum : Sum
  Sum1 : Sum
  Sum2 : Sum  Inputs=+-
  "abc -> dq (Power-Invariant)" : Subsystem  AncestorBlock=|
      | SimplusGT/abc -> dq
      | (Power-Invariant)
  w : Outport
  theta : Outport  Port=2
  idq : Outport  Port=3
  wires:
  Sum1/1 -> Math Function1/1
  Constant2/1 -> Sum1/2, [theta0]
  Math Function1/1 -> "abc -> dq (Power-Invariant)"/2(theta), [theta], theta/1
  Gain2/1 -> Sum/1
  Discrete-Time Integrator/1 -> Sum1/1
  Filter p/1 -> Sum2/2
  Constant/1 -> Sum/2
  "abc -> dq (Power-Invariant)"/1(dq) -> idq/1, Demux1/1
  Constant4/1 -> Math Function1/2
  iabc/1 -> "abc -> dq (Power-Invariant)"/1(abc)
  Gain1/1 -> Filter p/1
  Constant6/1 -> Sum2/1
  Sum2/1 -> Gain2/1
  Sum/1 -> Gain3/1
  Gain3/1 -> [w], w/1, Discrete-Time Integrator/1
  Demux1/1 -> Gain1/1, [id]  "id"
  Gain5/1 -> Scope/4
  [iq] -> Scope/2  "iq"
  [theta0] -> Mux/1  "theta"
  [id] -> Scope/1  "id"
  Mux/1 -> Gain5/1  "theta"
  [theta] -> Mux/2  "theta"
  Demux1/2 -> [iq]
  [w] -> Gain4/1  "w"
  Gain4/1 -> Scope/3

== system SimplusGT_2018b/Frequency Droop (iabc -> id+jiq) ==
  note: Measurement
  note: Frame trabsformation
  note: Current-frequency droop controller
      |
      | Author(s): Yitong Li
      |
      | Notes:
      |
      | The current reference should be in source convention.
      |
      | This droop controller controls both d- and q-axis currents.
  iabc : Inport
  Constant : Constant  Value=id0
  Constant10 : Constant  Value=theta_d0
  Constant2 : Constant  Value=wd0
  Constant4 : Constant  Value=2*pi
  Constant5 : Constant  Value=wq0
  Constant8 : Constant  Value=iq0
  Constant9 : Constant  Value=theta_q0
  Demux1 : Demux  Outputs=2
  Discrete-Time Integrator : DiscreteIntegrator  SampleTime=Ts  ICPrevOutput=DiscIntNeverNeededParam  ICPrevScaledInput=DiscIntNeverNeededParam
  Discrete-Time Integrator1 : DiscreteIntegrator  SampleTime=Ts  ICPrevOutput=DiscIntNeverNeededParam  ICPrevScaledInput=DiscIntNeverNeededParam
  Exp : Math  SaturateOnIntegerOverflow=on
  Filter p : DiscreteTransferFcn  Numerator=w_tau*Ts  Denominator=[1 ((w_tau*Ts)-1)]  SampleTime=Ts
  Filter p1 : DiscreteTransferFcn  Numerator=w_tau*Ts  Denominator=[1 ((w_tau*Ts)-1)]  SampleTime=Ts
  Gain : Gain  Gain=Wbase
  Gain1 : Gain  Gain=Wbase
  Gain2 : Gain  Gain=1/Wbase
  Gain4 : Gain  Gain=1/pi
  Gain5 : Gain  Gain=1/(Sbase/Vbase)
  Gain6 : Gain  Gain=m
  Gain7 : Gain  Gain=-1
  Gain8 : Gain  Gain=-1
  Gain9 : Gain  Gain=m
  Math Function1 : Math  Operator=mod  SaturateOnIntegerOverflow=on
  Mux : Mux  Inputs=2
  Mux1 : Mux  Inputs=2
  Mux2 : Mux  Inputs=2
  Product : Product
  Scope : Scope  NumInputPorts=3
  Sum : Sum  Inputs=|+-
  Sum{1..2,4..5} (4 alike) : Sum
  Sum3 : Sum  Inputs=|+-
  "abc -> dq (Power-Invariant)1" : Subsystem  AncestorBlock=|
      | SimplusGT/abc -> dq
      | (Power-Invariant)
  wd : Outport
  theta_d : Outport  Port=2
  wq : Outport  Port=3
  theta_q : Outport  Port=4
  wires:
  Gain2/1 -> Scope/2  "wdq"
  Discrete-Time Integrator/1 -> Sum5/1
  "abc -> dq (Power-Invariant)1"/1(dq) -> Gain5/1
  Math Function1/1 -> theta_d/1, [thetad]
  Mux2/1 -> Gain4/1  "thetadq"
  Constant5/1 -> Sum2/2
  Constant9/1 -> Sum4/2
  Gain5/1 -> Demux1/1
  Mux/1 -> Scope/1  "idq"
  Gain4/1 -> Scope/3  "thetadq"
  Demux1/2 -> [iq]
  Sum/1 -> Gain7/1
  Constant4/1 -> Math Function1/2
  Sum4/1 -> theta_q/1, [thetaq]
  Demux1/1 -> [id]
  Sum5/1 -> Math Function1/1
  Constant8/1 -> Sum3/2
  [wd] -> Mux1/1
  Constant/1 -> Sum/2
  [iq] -> Mux/2
  [thetaq] -> Mux2/2
  Mux1/1 -> Gain2/1  "wdq"
  Exp/1 -> Product/2
  [thetad] -> Mux2/1
  Constant2/1 -> Sum1/2
  [thetaq] -> Exp/1
  Constant10/1 -> Sum5/2
  [id] -> Mux/1
  Product/1 -> "abc -> dq (Power-Invariant)1"/1(abc)
  Discrete-Time Integrator1/1 -> Sum4/1
  Filter p/1 -> Sum3/1
  [thetad] -> "abc -> dq (Power-Invariant)1"/2(theta)
  [id] -> Filter p1/1
  iabc/1 -> Product/1
  [wq] -> Mux1/2
  [iq] -> Filter p/1
  Filter p1/1 -> Sum/1
  Gain9/1 -> Sum2/1
  Gain6/1 -> Sum1/1
  Gain7/1 -> Gain6/1
  Sum3/1 -> Gain8/1
  Gain8/1 -> Gain9/1
  Gain/1 -> [wd], wd/1, Discrete-Time Integrator/1
  Sum1/1 -> Gain/1
  Sum2/1 -> Gain1/1
  Gain1/1 -> [wq], wq/1, Discrete-Time Integrator1/1

== system SimplusGT_2018b/Frequency Droop (iabc -> iq) ==
  note: iq-frequency droop controller
      |
      | Author(s): Yitong Li
      |
      | Notes:
      |
      | The current reference should be in source convention.
      |
      | It is a iq-frequency droop controller rather than a power-frequency droop controller.
  note: Measurement
  iabc : Inport
  Constant : Constant  Value=w0
  Constant2 : Constant  Value=theta0
  Constant4 : Constant  Value=2*pi
  Constant6 : Constant  Value=i0
  Demux1 : Demux  Outputs=2
  Discrete-Time Integrator : DiscreteIntegrator  SampleTime=Ts  ICPrevOutput=DiscIntNeverNeededParam  ICPrevScaledInput=DiscIntNeverNeededParam
  Filter p : DiscreteTransferFcn  Numerator=w_tau*Ts  Denominator=[1 ((w_tau*Ts)-1)]  SampleTime=Ts
  Gain1 : Gain  Gain=1/(Sbase/Vbase)
  Gain2 : Gain  Gain=m
  Gain3 : Gain  Gain=Wbase
  Gain4 : Gain  Gain=1/Wbase
  Gain5 : Gain  Gain=1/pi
  Math Function1 : Math  Operator=mod  SaturateOnIntegerOverflow=on
  Mux : Mux  Inputs=2
  Scope : Scope  NumInputPorts=4
  Sum : Sum
  Sum1 : Sum
  Sum2 : Sum  Inputs=+-
  "abc -> dq (Power-Invariant)1" : Subsystem  AncestorBlock=|
      | SimplusGT/abc -> dq
      | (Power-Invariant)
  w : Outport
  theta : Outport  Port=2
  idq : Outport  Port=3
  wires:
  Demux1/2 -> Gain1/1, [iq]
  Sum1/1 -> Math Function1/1
  Gain3/1 -> Discrete-Time Integrator/1, [w], w/1
  Filter p/1 -> Sum2/2
  Constant6/1 -> Sum2/1
  Gain1/1 -> Filter p/1
  Discrete-Time Integrator/1 -> Sum1/1
  Constant2/1 -> [theta0], Sum1/2
  Sum2/1 -> Gain2/1
  Sum/1 -> Gain3/1
  Constant/1 -> Sum/2
  "abc -> dq (Power-Invariant)1"/1(dq) -> idq/1, Demux1/1
  Constant4/1 -> Math Function1/2
  Math Function1/1 -> [theta], theta/1, "abc -> dq (Power-Invariant)1"/2(theta)
  Gain2/1 -> Sum/1
  iabc/1 -> "abc -> dq (Power-Invariant)1"/1(abc)
  [iq] -> Scope/2  "iq"
  Mux/1 -> Gain5/1
  [theta0] -> Mux/1  "theta"
  [id] -> Scope/1  "id"
  Gain5/1 -> Scope/4
  [theta] -> Mux/2  "theta"
  Demux1/1 -> [id]  "id"
  Gain4/1 -> Scope/3
  [w] -> Gain4/1  "w"

== system SimplusGT_2018b/Grid-Feeding Buck (System Object) ==
  note: Matlab System Object
  note: Auxiliary
  note: Electrical Circuit
  note: Grid-feeding buck dc-dc converter.
      |
      | Author(s): Yitong Li
      |
      | Notes:
      |
      | The model is based on matlab system object.
      |
      | The model is in load convention.
  Bus Creator : BusCreator  Inputs=4
  Constant : Constant  Value=OtherInputs
  Current Measurement : powerlib/Measurements/Current Measurement  PhasorSimulation=off  OutputType=Complex  PSBequivalent=0
  Demux : Demux  Outputs=2
  Gain1 : Gain  Gain=1/Vbase
  Gain2 : Gain  Gain=Sbase/Vbase
  Gain3 : Gain  Gain=1/(Sbase/Vbase)
  MATLAB System1 : MATLABSystem  System=SimplusGT.Class.GridFeedingBuck  Ts=Ts  Para=ApparatusPara  ApparatusType=ApparatusType  PowerFlow=PowerFlow  x0=x0  DiscreMethod=DiscreMethod  LinearizationTimes=LinearizationTimes  DirectFeedthrough=DirectFeedthrough  VirtualResistor=DiscreDampingFlag  EquiInitial=true  ElecPortIOs=[1]  SimulateUsing=Code generation
      mask Type: SimplusGT.Class.GridFeedingBuck
      mask Display:
      | disp('GridFeedingBuck');
      | port_label('input',1,'u');
      | port_label('output',1,'y');
  Mux2 : Mux  Inputs=2
  Product : Product
  R_VD : powerlib/Elements/Series RLC Branch  LConnTagsString=__new0  RConnTagsString=__new0  BranchType=R  Resistance=DiscreDampingValue*Vbase^2/Sbase  Inductance=1e-3  SetiL0=off  InitialCurrent=0  Capacitance=1e-6  Setx0=off  InitialVoltage=0  Measurements=None
  ia : powerlib/Electrical Sources/Controlled Current Source  Initialize=on  Source_Type=AC  Amplitude=0  Phase=0  Frequency=0  Measurements=None
  v : powerlib/Measurements/Voltage Measurement  PhasorSimulation=off  OutputType=Complex  PSBequivalent=0
  a : PMIOPort  Side=Left
  b : PMIOPort  Port=2  Side=Left
  m : Outport
  wires:
  Gain2/1 -> ia/1
  v/1 -> Gain1/1
  [v] -> Mux2/1
  [v] -> Bus Creator/1  "v"
  Gain1/1 -> [v]
  Demux/1 -> [i]
  Mux2/1 -> MATLAB System1/1
  MATLAB System1/1 -> Demux/1
  Demux/2 -> [v_dc]
  Bus Creator/1 -> m/1
  [i] -> Gain2/1
  Product/1 -> [p]
  Constant/1 -> Mux2/2
  [v] -> Product/1  "v"
  [i_t] -> Product/2  "i"
  [i_t] -> Bus Creator/2  "i"
  [p] -> Bus Creator/3  "p"
  [v_dc] -> Bus Creator/4  "v_dc"
  Current Measurement/1 -> Gain3/1
  Gain3/1 -> [i_t]
  connections:
  b/RConn1 -- v/LConn2 -- ia/RConn1 -- R_VD/RConn1
  R_VD/LConn1 -- Current Measurement/RConn1 -- v/LConn1 -- ia/LConn1
  Current Measurement/LConn1 -- a/RConn1
